simulink model "ex2inicio"  (R2012b)
settings: Solver=ode45  StartTime=0.0  StopTime=10.0  RelTol=1e-9
undefined symbols (not defined in the file or in its folder): heaviside, sigbuilder_block
settings Model: Creator=Katarina  LastModifiedBy=Katarina
settings DataIOCC: LimitDataPoints=off
settings DebuggingCC: SolverPrmCheckMsg=none

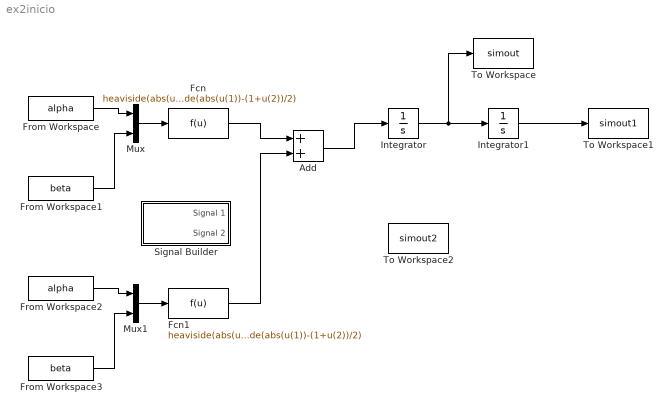
== system ex2inicio ==
  Add : Sum
  Fcn : Fcn  Expr=heaviside(abs(u(1)))-0.5*heaviside(abs(u(1))-(1-u(2))/2)-0.5*heaviside(abs(u(1))-(1+u(2))/2)
  Fcn1 : Fcn  Expr=heaviside(abs(u(1)))-0.5*heaviside(abs(u(1))-(1-u(2))/2)-0.5*heaviside(abs(u(1))-(1+u(2))/2)
  From Workspace : FromWorkspace  VariableName=alpha  SampleTime=0
  From Workspace1 : FromWorkspace  VariableName=beta  SampleTime=0
  From Workspace2 : FromWorkspace  VariableName=alpha  SampleTime=0
  From Workspace3 : FromWorkspace  VariableName=beta  SampleTime=0
  Integrator : Integrator
  Integrator1 : Integrator
  Mux : Mux  Inputs=2
  Mux1 : Mux  Inputs=2
  Signal Builder : Subsystem  Tag=STV Subsys  LoadFcn=sigbuilder_block('load');  StartFcn=sigbuilder_block('start');  StopFcn=sigbuilder_block('stop');  ClipboardFcn=sigbuilder_block('clipboard');  mask(Sigbuilder block){}
      mask help: Simulink:masks:SigbuilderBlock_MD
      mask init:
      | if ~strcmp(get_param(bdroot(gcbh),'SimulationStatus'),'stopped') tuvar = sigbuilder_block('maskInit'); end
      settings: CopyFcn=sigbuilder_block('copy');  DeleteFcn=sigbuilder_block('delete');  ModelCloseFcn=sigbuilder_block('modelClose');  PreSaveFcn=sigbuilder_block('preSave');  PauseFcn=sigbuilder_block('pause');  ContinueFcn=sigbuilder_block('continue');  NameChangeFcn=sigbuilder_block('namechange');  OpenFcn=sigbuilder_block('open',[440.25 121.5 544.5 391.5 ]);  CloseFcn=sigbuilder_block('close');
      mask Display: plot(0, 0, 100, 100,[2, 2, 32, 32, 2], [68, 8, 8, 68, 68],[32, 2], [38, 38], [32, 19, 2],[53, 60, 44], [32, 17, 17, 2],[16, 16, 31, 31]);txt = getActiveGroup(gcbh);text(2, 100, txt,'verticalAlignment', 'top');
  To Workspace : ToWorkspace  VariableName=simout  SampleTime=-1  SaveFormat=Timeseries
  To Workspace1 : ToWorkspace  VariableName=simout1  SampleTime=-1  SaveFormat=Timeseries
  To Workspace2 : ToWorkspace  VariableName=simout2  SampleTime=-1  SaveFormat=Timeseries
  wires:
  From Workspace/1 -> Mux/1
  From Workspace1/1 -> Mux/2
  Mux/1 -> Fcn/1
  Integrator/1 -> To Workspace/1, Integrator1/1
  Integrator1/1 -> To Workspace1/1
  From Workspace2/1 -> Mux1/1
  From Workspace3/1 -> Mux1/2
  Mux1/1 -> Fcn1/1
  Fcn1/1 -> Add/2
  Fcn/1 -> Add/1
  Add/1 -> Integrator/1

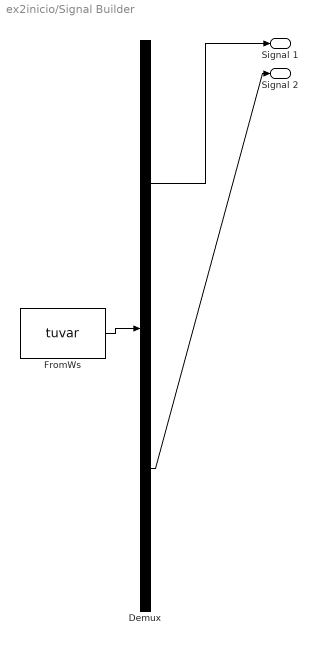
== system ex2inicio/Signal Builder ==
  Demux : Demux  Tag=STV Demux  Outputs=2
  FromWs : FromWorkspace  Tag=STV FromWs  VariableName=tuvar  SampleTime=0
      SigBuilderData=|
      | common.afterFinalStr = 'Extrapolate'
      | common.sampleTime = 0
      | dataSet.timeRange = [0 10]
      | dataSet.name = 'Group 1'
      | sbobj.Groups.Name = 'Group 1'
      | sbobj.Groups.Signals(1).Name = 'Signal 1'
      | sbobj.Groups.Signals(1).XData = [0 4 4 6 6 10]
      | sbobj.Groups.Signals(1).YData = [0 0 1 1 0 0]
      | sbobj.Groups.Signals(2).Name = 'Signal 2'
      | sbobj.Groups.Signals(2).XData = [0 4 4 6 6 10]
      | sbobj.Groups.Signals(2).YData = [0 0 1 1 0 0]
  Signal 1 : Outport  Tag=STV Outport
  Signal 2 : Outport  Tag=STV Outport  Port=2
  wires:
  Demux/1 -> Signal 1/1
  FromWs/1 -> Demux/1
  Demux/2 -> Signal 2/1
